simulink model "Sampling_Theorem"  (R2021a)
settings: Solver=VariableStepAuto  StartTime=0.0  StopTime=0.01  RelTol=1e-3
settings Model: Creator=Mrittik  LastModifiedBy=Mrittik

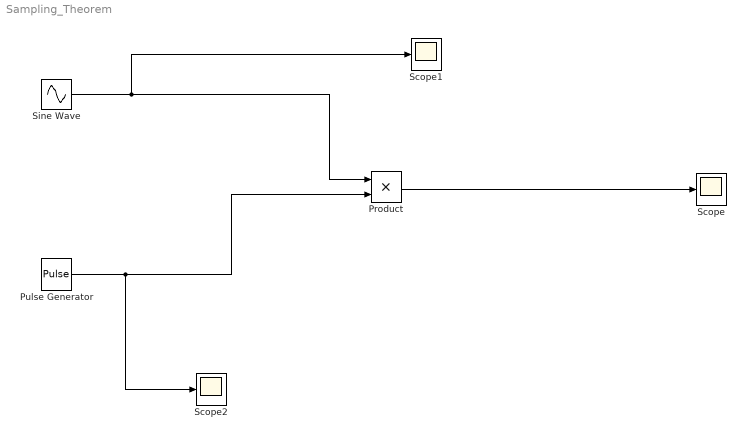
== system Sampling_Theorem ==
  Product : Product
  Pulse Generator : DiscretePulseGenerator  PulseType=Time based  Amplitude=2  Period=1/2000  PulseWidth=50
  Scope : Scope
  Scope1 : Scope
  Scope2 : Scope
  Sine Wave : Sin  Amplitude=2  Frequency=1000  SampleTime=0
  wires:
  Sine Wave/1 -> Scope1/1, Product/1
  Pulse Generator/1 -> Scope2/1, Product/2
  Product/1 -> Scope/1
